simulink model "pll_d0_fncd"  (Simulink 7.4)
settings: Solver=ode45  StartTime=0.0  StopTime=1e-4  MaxStep=1/(4*5e6)  RelTol=1e-1
PreLoadFcn:
  | k0=1; k1= 1; k2 =1; k3=1; k4=1;
libraries: simulink_extras x2, dsparch4 x1, simulink x1, sdolib x1, commsynccomp2 x1
settings Model: Creator=dbenson  LastModifiedBy=Dick  ExtModeTrigMode=oneshot  ExtModeArmWhenConnect=off  BufferReuse=off
settings DataIOCC: LimitDataPoints=off  SaveOutput=off  SaveTime=off
settings OptimizationCC: BooleanDataType=off  InlineInvariantSignals=on  OptimizeBlockIOStorage=off  BufferReuse=off  ExpressionFolding=off  LocalBlockOutputs=off  InitFltsAndDblsToZero=on
settings DebuggingCC: SaveWithParameterizedLinksMsg=none  SignalResolutionControl=TryResolveAllWithWarning  SolverPrmCheckMsg=none  MultiTaskDSMMsg=warning  MultiTaskCondExecSysMsg=none  StrictBusMsg=None
settings HardwareCC: TargetUnknown=on
settings RTWCC: IncludeERTFirstTime=on
settings GRTTargetCC: TargetFcnLib=ansi_tfl_tmw.mat

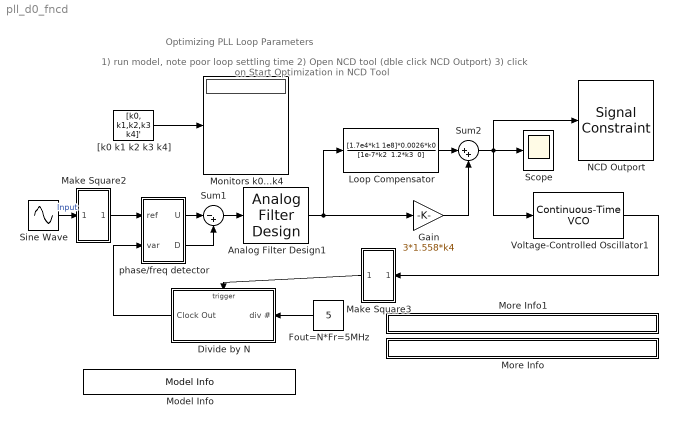
== system pll_d0_fncd ==
  note: 1) run model, note poor loop settling time
      | 2) Open NCD tool (dble click NCD Outport)
      | 3) click on Start Optimization in NCD Tool
  note: Optimizing PLL Loop Parameters
  Analog Filter Design1 : dsparch4/Analog Filter Design  method=Elliptic  filttype=Lowpass  N=4  Wlo=2*pi*350e3  Whi=80  Rp=3  Rs=80
  Divide by N : Subsystem  AncestorBlock=rab_favorites/Divide by N  TreatAsAtomicUnit=on
  Fout=N*Fr=5MHz : Constant  Value=5  OutDataType=sfix(16)  OutScaling=2^0
  Gain : Gain  Gain=3*1.558*k4  ParameterDataType=sfix(16)  ParameterScaling=2^0  OutDataType=sfix(16)  OutScaling=2^0  SaturateOnIntegerOverflow=on  OutDataTypeStr=Inherit: Same as input  ParamDataTypeStr=Inherit: Same as input
  Loop Compensator : TransferFcn  Numerator=[1.7e4*k1 1e8]*0.0026*k0  Denominator="[1e-7*k2  1.2*k3  0]"
  Make Square2 : Subsystem
      mask Type: Make Square
      mask Description:
      | For input +ve values output is 1
      | For input -ve values output is 0
      mask Display: plot(0,0,100,100,[90,70,70,50,50,30,30,10,10],[20,20,40,40,20,20,40,40,20],[90,87,84,80,76,73,70,67,63,60,57,53,50,47,44,40,36,33,30,27,23,20,17,13,10],[70,65,63,62,63,65,70,75,77,78,77,75,70,65,63,62,63,65,70,75,77,78,77,75,70])
  Make Square3 : Subsystem
      mask Type: Make Square
      mask Description:
      | For input +ve values output is 1
      | For input -ve values output is 0
      mask Display: plot(0,0,100,100,[90,70,70,50,50,30,30,10,10],[20,20,40,40,20,20,40,40,20],[90,87,84,80,76,73,70,67,63,60,57,53,50,47,44,40,36,33,30,27,23,20,17,13,10],[70,65,63,62,63,65,70,75,77,78,77,75,70,65,63,62,63,65,70,75,77,78,77,75,70])
  Model Info : simulink/Model-Wide Utilities/Model Info  SystemSampleTime=-1  InitialBlockCM=none  BlockCM=none  Frame=on  DisplayStringWithTags=Copywrite 2005-2010 The MathWorks, Inc.  HorizontalTextAlignment=Center  LeftAlignmentValue=0.5  SourceBlockDiagram=pll_d0_fncd  TagMaxNumber=20
  "Monitors k0...k4 " : Display
  More Info : Subsystem  AncestorBlock=rab_favorites/More Info
      settings: OpenFcn=k0=1; k1=1; k2=1; k3=1; k4=1;
      mask Display: disp('double click to restore initial k0 k1 k2 k3 k4 values')
  More Info1 : Subsystem  AncestorBlock=rab_favorites/More Info
      settings: OpenFcn=k0=0.2623; k1=2.625; k2=2.54; k3=3.775; k4=2.202;
      mask Display: disp('double click to restore OPTIMAL k0 k1 k2 k3 k4 values')
  NCD Outport : sdolib/Signal Constraint  SystemSampleTime=-1  DialogPosition=[0.294375 0.147777777777778 0.45 0.31]  SaveIn=MAT file  SaveAs=pll_d0_fncd_optim.mat  LogID=SRO_DataLog_1
  Scope : Scope
      settings: TimeRange=0.00012  YMin=-0.2  YMax=1.4
  Sine Wave : Sin  Amplitude=1  Bias=0  Frequency=2*pi*(1e6)  Phase=pi  Samples=10  SampleTime=0  Offset=0
  Sum1 : Sum  Inputs=|-+  OutDataType=sfix(16)  OutScaling=2^0  SaturateOnIntegerOverflow=on  InputSameDT=on  OutDataTypeStr=Inherit: Same as first input
  Sum2 : Sum  Inputs=|++  OutDataType=sfix(16)  OutScaling=2^0  SaturateOnIntegerOverflow=on  InputSameDT=on  OutDataTypeStr=Inherit: Same as first input
  Voltage-Controlled Oscillator1 : commsynccomp2/Continuous-Time VCO  SystemSampleTime=-1  Ac=1  Fc=4.9e6  Kc=0.1e6  Ph=pi*0.6
  "[k0 k1 k2 k3 k4]" : Constant  Value=[k0, k1,k2,k3 k4]'  VectorParams1D=off  OutDataType=sfix(16)  OutScaling=2^0
  phase/freq detector : Subsystem
  wires:
  Sine Wave/1 -> Make Square2/1(In1)  "Input"
  Voltage-Controlled Oscillator1/1 -> Make Square3/1(In1)
  Make Square2/1(Out1) -> phase/freq detector/1(ref)
  phase/freq detector/1(U) -> Sum1/1
  phase/freq detector/2(D) -> Sum1/2
  Sum1/1 -> Analog Filter Design1/1
  Make Square3/1(Out1) -> Divide by N/Trigger
  Fout=N*Fr=5MHz/1 -> Divide by N/1(div #)
  Divide by N/1(Clock Out) -> phase/freq detector/2(var)
  "[k0 k1 k2 k3 k4]"/1 -> "Monitors k0...k4 "/1
  Loop Compensator/1 -> Sum2/1
  Gain/1 -> Sum2/2
  Sum2/1 -> NCD Outport/1, Scope/1, Voltage-Controlled Oscillator1/1
  Analog Filter Design1/1 -> Loop Compensator/1, Gain/1

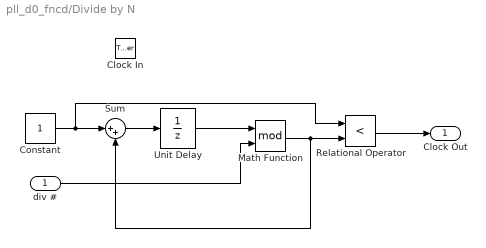
== system pll_d0_fncd/Divide by N ==
  div # : Inport  OutDataType=sfix(16)  OutScaling=2^0
  Clock In : TriggerPort
  Constant : Constant  OutDataType=sfix(16)  OutScaling=2^0
  Math Function : Math  Operator=mod  OutDataType=sfix(16)  OutScaling=2^0  SaturateOnIntegerOverflow=on
  Relational Operator : RelationalOperator  Operator=<  InputSameDT=on
  Sum : Sum  Inputs=|++  OutDataType=sfix(16)  OutScaling=2^0  SaturateOnIntegerOverflow=on  InputSameDT=on  OutDataTypeStr=Inherit: Same as first input
  Unit Delay : UnitDelay  SampleTime=-1
  Clock Out : Outport  OutDataType=sfix(16)  OutScaling=2^0
  wires:
  Constant/1 -> Sum/1, Relational Operator/1
  Sum/1 -> Unit Delay/1
  Unit Delay/1 -> Math Function/1
  div #/1 -> Math Function/2
  Math Function/1 -> Sum/2, Relational Operator/2
  Relational Operator/1 -> Clock Out/1

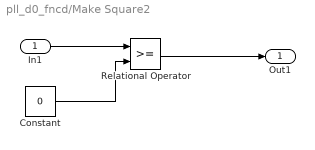
== system pll_d0_fncd/Make Square2 ==
  In1 : Inport  OutDataType=sfix(16)  OutScaling=2^0
  Constant : Constant  Value=0  OutDataType=sfix(16)  OutScaling=2^0
  Relational Operator : RelationalOperator  InputSameDT=on
  Out1 : Outport  OutDataType=sfix(16)  OutScaling=2^0
  wires:
  Relational Operator/1 -> Out1/1
  Constant/1 -> Relational Operator/2
  In1/1 -> Relational Operator/1

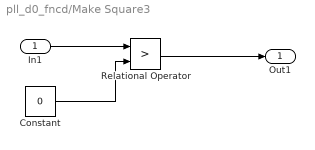
== system pll_d0_fncd/Make Square3 ==
  In1 : Inport  OutDataType=sfix(16)  OutScaling=2^0
  Constant : Constant  Value=0  OutDataType=sfix(16)  OutScaling=2^0
  Relational Operator : RelationalOperator  Operator=>  InputSameDT=on
  Out1 : Outport  OutDataType=sfix(16)  OutScaling=2^0
  wires:
  In1/1 -> Relational Operator/1
  Constant/1 -> Relational Operator/2
  Relational Operator/1 -> Out1/1

== system pll_d0_fncd/More Info ==
  note: This is an "info" block

== system pll_d0_fncd/More Info1 ==
  note: This is an "info" block

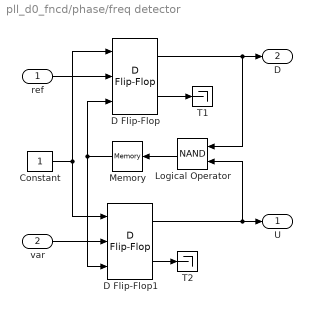
== system pll_d0_fncd/phase/freq detector ==
  ref : Inport  OutDataType=sfix(16)  OutScaling=2^0
  var : Inport  Port=2  OutDataType=sfix(16)  OutScaling=2^0
  Constant : Constant  OutDataType=sfix(16)  OutScaling=2^0
  D Flip-Flop : simulink_extras/Flip Flops/D Flip-Flop  SystemSampleTime=-1
  D Flip-Flop1 : simulink_extras/Flip Flops/D Flip-Flop  SystemSampleTime=-1
  Logical Operator : Logic  Operator=NAND
  Memory : Memory
  T1 : Terminator
  T2 : Terminator
  U : Outport  OutDataType=sfix(16)  OutScaling=2^0
  D : Outport  Port=2  OutDataType=sfix(16)  OutScaling=2^0
  wires:
  ref/1 -> D Flip-Flop/2
  var/1 -> D Flip-Flop1/2
  Constant/1 -> D Flip-Flop/1, D Flip-Flop1/1
  Logical Operator/1 -> Memory/1
  Memory/1 -> D Flip-Flop/3, D Flip-Flop1/3
  D Flip-Flop/1 -> Logical Operator/1, D/1
  D Flip-Flop1/1 -> Logical Operator/2, U/1
  D Flip-Flop/2 -> T1/1
  D Flip-Flop1/2 -> T2/1
